simulink model "CoreNozzletst"  (R2025a)
settings: Solver=VariableStepAuto  StartTime=0.0  StopTime=10.0  RelTol=1e-3
settings Model: Creator=ramch  LastModifiedBy=ramch

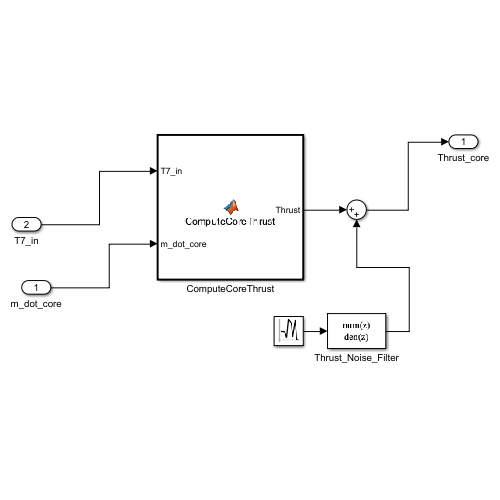
[thumbnail: Simulink's stored preview of the top-level diagram]
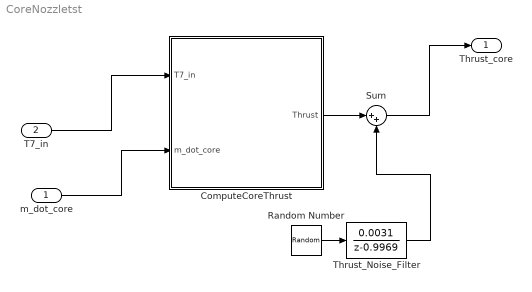
== system CoreNozzletst ==
  m_dot_core : Inport
  T7_in : Inport  Port=2
  ComputeCoreThrust : MATLAB Function  TreatAsAtomicUnit=on
  Random Number : RandomNumber  Variance=500  SampleTime=0.001
  Sum : Sum  Inputs=|++
  Thrust_Noise_Filter : DiscreteTransferFcn  Numerator=0.0031  Denominator=1 -0.9969  InitialStates=0.001
  Thrust_core : Outport
  wires:
  T7_in/1 -> ComputeCoreThrust/1(T7_in)
  m_dot_core/1 -> ComputeCoreThrust/2(m_dot_core)
  ComputeCoreThrust/1(Thrust) -> Sum/1
  Sum/1 -> Thrust_core/1
  Thrust_Noise_Filter/1 -> Sum/2
  Random Number/1 -> Thrust_Noise_Filter/1

== matlab function CoreNozzletst/ComputeCoreThrust ==
  data: T7_in input; Thrust output; m_dot_core input
function Thrust = ComputeCoreThrust(T7_in, m_dot_core)
    cp = 1150;           % J/kg·K (core gas specific heat)
    T_ambient = 288;     % K (standard sea level)
    V_ambient = 0;       % m/s (static case)
    
    % Ensure physical realism
    if T7_in > T_ambient
        V_exit = sqrt(2 * cp * (T7_in - T_ambient));
    else
        V_exit = 0;
    end

    Thrust = m_dot_core * (V_exit - V_ambient);
end
